simulink model "Suspension_simulink_simscape"  (R2024a)
settings: Solver=FixedStepAuto  StartTime=0.0  StopTime=10  FixedStep=0.00001  RelTol=1e-3
InitFcn:
  | m1 = 290;
  | m2 = 59;
  | b1 = 1000;
  | k1 = 16182;
  | k2 = 19000;
  | f = 0;
libraries: fl_lib x10, nesl_utility x7
settings Model: Creator=USUARIO  LastModifiedBy=USUARIO

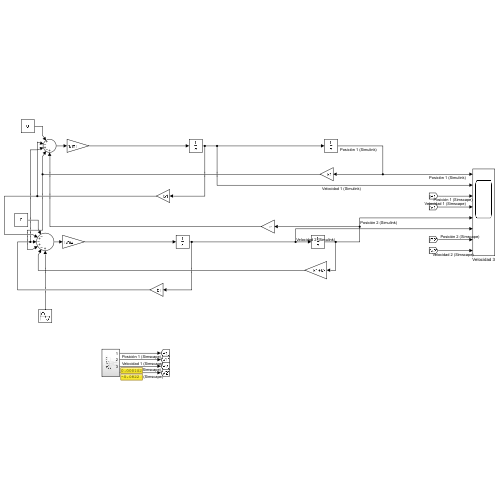
[thumbnail: Simulink's stored preview of the top-level diagram]
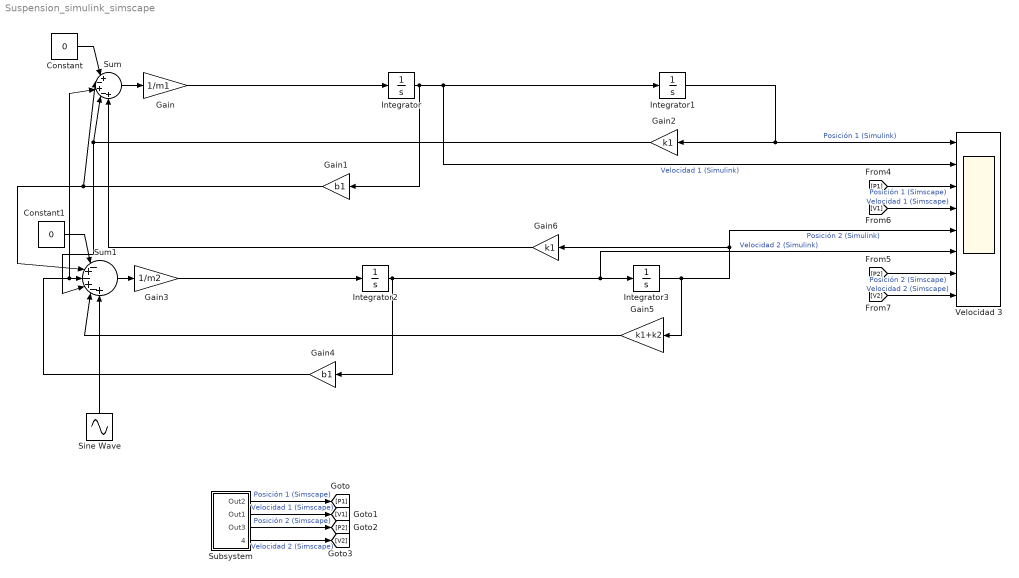
== system Suspension_simulink_simscape ==
  Constant : Constant  Value=0
  Constant1 : Constant  Value=0
  Gain : Gain  Gain=1/m1
  Gain1 : Gain  Gain=b1
  Gain2 : Gain  Gain=k1
  Gain3 : Gain  Gain=1/m2
  Gain4 : Gain  Gain=b1
  Gain5 : Gain  Gain=k1+k2
  Gain6 : Gain  Gain=k1
  Integrator{,1..3} (4 alike) : Integrator
  Sine Wave : Sin  Amplitude=0.05*k2  Frequency=0.5*pi  SampleTime=0
  Subsystem : Subsystem
  Sum : Sum  Inputs=|+-+-+
  Sum1 : Sum  Inputs=|-+-+-+
  Velocidad 3 : Scope  NumInputPorts=8
  wires:
  Constant/1 -> Sum/1
  Sum/1 -> Gain/1
  Integrator/1 -> Gain1/1, Velocidad 3/2, Integrator1/1  "Velocidad 1 (Simulink)"
  Gain/1 -> Integrator/1
  Integrator1/1 -> Velocidad 3/1, Gain2/1  "Posición 1 (Simulink)"
  Gain1/1 -> Sum1/2, Sum/2
  Gain2/1 -> Sum1/4, Sum/4
  Gain5/1 -> Sum1/5
  Gain4/1 -> Sum/3, Sum1/3
  Integrator3/1 -> Velocidad 3/5, Gain6/1, Gain5/1  "Posición 2 (Simulink)"
  Gain3/1 -> Integrator2/1
  Integrator2/1 -> Velocidad 3/6, Integrator3/1, Gain4/1  "Velocidad 2 (Simulink)"
  Sum1/1 -> Gain3/1
  Constant1/1 -> Sum1/1
  Sine Wave/1 -> Sum1/6
  Gain6/1 -> Sum/5
  Subsystem/4(4) -> [V2]  "Velocidad 2 (Simscape)"
  Subsystem/3(Out3) -> [P2]  "Posición 2 (Simscape)"
  Subsystem/2(Out1) -> [V1]  "Velocidad 1 (Simscape)"
  Subsystem/1(Out2) -> [P1]  "Posición 1 (Simscape)"
  [P1] -> Velocidad 3/3  "Posición 1 (Simscape)"
  [V1] -> Velocidad 3/4  "Velocidad 1 (Simscape)"
  [P2] -> Velocidad 3/7  "Posición 2 (Simscape)"
  [V2] -> Velocidad 3/8  "Velocidad 2 (Simscape)"

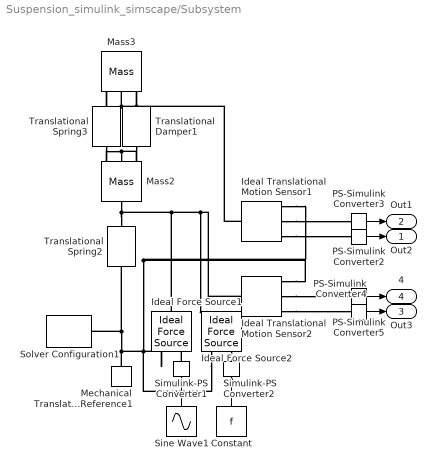
== system Suspension_simulink_simscape/Subsystem ==
  Constant : Constant  Value=f
  Ideal Force Source1 : fl_lib/Mechanical/Mechanical Sources/Ideal Force Source
  Ideal Force Source2 : fl_lib/Mechanical/Mechanical Sources/Ideal Force Source
  Ideal Translational Motion Sensor1 : fl_lib/Mechanical/Mechanical Sensors/Ideal Translational Motion Sensor  reference=foundation.enum.MeasurementReference.difference  acceleration_port=false  velocity_port=true  position_port=true  offset=0 m
  Ideal Translational Motion Sensor2 : fl_lib/Mechanical/Mechanical Sensors/Ideal Translational Motion Sensor  reference=foundation.enum.MeasurementReference.difference  acceleration_port=false  velocity_port=true  position_port=true  offset=0 m
  Mass2 : fl_lib/Mechanical/Translational Elements/Mass  mass=m2 kg  num_ports=foundation.enum.numPorts2.two  v_specify=off  v_priority=High  v=0 m/s  v_nominal_specify=off  v_nominal_value=1  v_nominal_unit=m/s  f_specify=off  f_priority=None  f=0 N  f_nominal_specify=off  f_nominal_value=1  f_nominal_unit=N
      settings: InternalSimscapePortConfiguration="{\"Bottom\":[],\"Left\":[{\"id\":\"M\",\"label\":\"\",\"type\":\"foundation.mechanical.translational.translational\"}],\"Right\":[{\"id\":\"N\",\"label\":\"\",\"type\":\"foundation.mechanical.translational.translational\"}],\"Top\":[]}"
  Mass3 : fl_lib/Mechanical/Translational Elements/Mass  mass=m1 kg  num_ports=foundation.enum.numPorts2.one  v_specify=off  v_priority=High  v=0 m/s  v_nominal_specify=off  v_nominal_value=1  v_nominal_unit=m/s  f_specify=off  f_priority=None  f=0 N  f_nominal_specify=off  f_nominal_value=1  f_nominal_unit=N
  Mechanical Translational Reference1 : fl_lib/Mechanical/Translational Elements/Mechanical Translational Reference
  PS-Simulink Converter{2..5} (4 alike) : nesl_utility/PS-Simulink Converter  PhysicalDomain=network_engine_domain  SubClassName=ps_output  LeftPortType=input  RightPortType=output  PseudoPeriodic=off  Frequencies=[]  VectorFormat=inherit  Unit=inherit  AffineConversion=off
  Simulink-PS Converter1 : nesl_utility/Simulink-PS Converter  PhysicalDomain=network_engine_domain  SubClassName=ps_input  LeftPortType=input  RightPortType=output  PseudoPeriodic=off  Frequencies=[]  NoiseDistribution=none  NoiseParameters=[]  Unit=1  AffineConversion=off  FilteringAndDerivatives=provide  SimscapeFilterOrder=1  InputFilterTimeConstant=0.001  UdotUserProvided=0
  Simulink-PS Converter2 : nesl_utility/Simulink-PS Converter  PhysicalDomain=network_engine_domain  SubClassName=ps_input  LeftPortType=input  RightPortType=output  PseudoPeriodic=off  Frequencies=[]  NoiseDistribution=none  NoiseParameters=[]  Unit=1  AffineConversion=off  FilteringAndDerivatives=provide  SimscapeFilterOrder=1  InputFilterTimeConstant=0.001  UdotUserProvided=0
  Sine Wave1 : Sin  Amplitude=0.05*k2  Frequency=0.5*pi  SampleTime=0
  Solver Configuration1 : nesl_utility/Solver Configuration  PhysicalDomain=network_engine_domain  SubClassName=solver  LeftPortType=input  RightPortType=generic  Tones=[]  Harmonics=[]  SimulateNoise=off  Profile=off  UseLocalSampling=off  EnableSwitchedLinearOptims=on  FrequencyDomain=off  UseCCode=off  RelTol=0.001  AbsTol=0.001  MinStep=1e-09  ToWorkspace=off  RevertToSquareIcSolve=off  NumHomotopyIterations=100  PhasorMode=off  PhasorModeNumHarmonics=1  ConsistencySolver=NEWTON_XTOL_AFTER_FTOL  IndexReductionMethod=DerivativeReplacement  DoDC=off  ResidualTolerance=1e-09  ConsistencyTolSource=GLOBAL  ConsistencyAbsTol=0.001  ConsistencyRelTol=0.001  ConsistencyTolFactor=0.000001  UseLocalSolver=off  LocalSolverChoice=NE_BACKWARD_EULER_ADVANCER  ResolveIndetEquations=on  FunctionEvalNumThread=1  LocalSolverSampleTime=0.001  DoFixedCost=off  MaxNonlinIter=3  MaxModeIter=2  ComputeImpulses=off  ImpulseIterations=2  LinearAlgebra=auto  LinearAlgebraNumThread=0  EquationFormulation=NE_TIME_EF  DelaysMemoryBudget=1024  AutomaticFiltering=on  FilteringTimeConstant=0.001  PartitionStorageMethod=AS_NEEDED  PartitionMemoryBudget=1024  PartitionMethod=ROBUST  MultibodyUseLocalSolver=off  MultibodyLocalSolverChoice=ODE1  MultibodyLocalSolverSampleTime=0.001
  Translational Damper1 : fl_lib/Mechanical/Translational Elements/Translational Damper  D=b1 N*s/m  v_specify=off  v_priority=None  v=0 m/s  v_nominal_specify=off  v_nominal_value=1  v_nominal_unit=m/s  f_specify=off  f_priority=None  f=0 N  f_nominal_specify=off  f_nominal_value=1  f_nominal_unit=N
  Translational Spring2 : fl_lib/Mechanical/Translational Elements/Translational Spring  spr_rate=k2 N/m  v_specify=off  v_priority=None  v=0 m/s  v_nominal_specify=off  v_nominal_value=1  v_nominal_unit=m/s  f_specify=off  f_priority=None  f=0 N  f_nominal_specify=off  f_nominal_value=1  f_nominal_unit=N  x_specify=off  x_priority=High  x=0 m  x_nominal_specify=off  x_nominal_value=1  x_nominal_unit=m
  Translational Spring3 : fl_lib/Mechanical/Translational Elements/Translational Spring  spr_rate=k1 N/m  v_specify=off  v_priority=None  v=0 m/s  v_nominal_specify=off  v_nominal_value=1  v_nominal_unit=m/s  f_specify=off  f_priority=None  f=0 N  f_nominal_specify=off  f_nominal_value=1  f_nominal_unit=N  x_specify=off  x_priority=High  x=0 m  x_nominal_specify=off  x_nominal_value=1  x_nominal_unit=m
  Out2 : Outport
  Out1 : Outport  Port=2
  Out3 : Outport  Port=3
  4 : Outport  Port=4
  wires:
  Sine Wave1/1 -> Simulink-PS Converter1/1
  PS-Simulink Converter5/1 -> 4/1
  PS-Simulink Converter2/1 -> Out2/1
  PS-Simulink Converter3/1 -> Out1/1
  PS-Simulink Converter4/1 -> Out3/1
  Constant/1 -> Simulink-PS Converter2/1
  connections:
  Translational Damper1/LConn1 -- Ideal Translational Motion Sensor1/LConn1 -- Mass3/LConn1 -- Translational Spring3/LConn1
  Translational Damper1/RConn1 -- Mass2/RConn1 -- Translational Spring3/RConn1
  Mechanical Translational Reference1/LConn1 -- Ideal Force Source2/RConn2 -- Ideal Translational Motion Sensor2/RConn1 -- Ideal Translational Motion Sensor1/RConn1 -- Ideal Force Source1/RConn2 -- Translational Spring2/RConn1 -- Solver Configuration1/RConn1
  Mass2/LConn1 -- Ideal Translational Motion Sensor2/LConn1 -- Ideal Force Source2/LConn1 -- Ideal Force Source1/LConn1 -- Translational Spring2/LConn1
  Simulink-PS Converter1/RConn1 -- Ideal Force Source1/RConn1
  Ideal Translational Motion Sensor2/RConn2 -- PS-Simulink Converter5/LConn1
  Ideal Translational Motion Sensor2/RConn3 -- PS-Simulink Converter4/LConn1
  Ideal Translational Motion Sensor1/RConn2 -- PS-Simulink Converter3/LConn1
  Ideal Translational Motion Sensor1/RConn3 -- PS-Simulink Converter2/LConn1
  Ideal Force Source2/RConn1 -- Simulink-PS Converter2/RConn1
